simulink model "Ex4"  (R2022a)
settings: Solver=FixedStepAuto  StartTime=0.0  StopTime=5  FixedStep=0.1  RelTol=1e-3
undefined symbols (not defined in the file or in its folder): ThetaA0, XdotC0
settings Model: Creator=vfton  LastModifiedBy=vfton

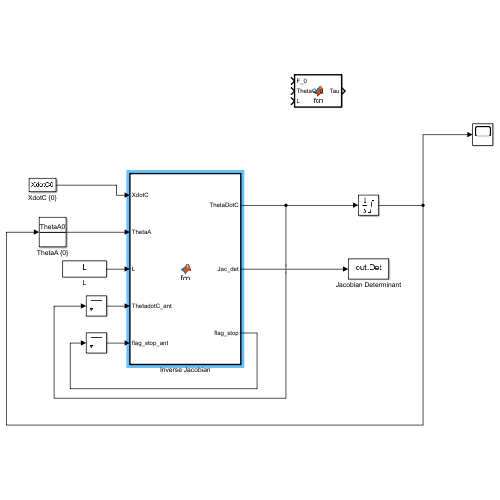
[thumbnail: Simulink's stored preview of the top-level diagram]
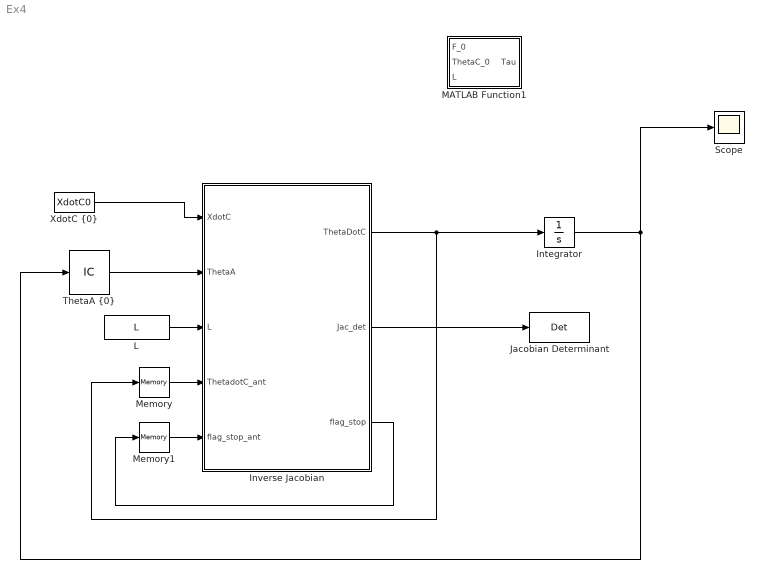
== system Ex4 ==
  Integrator : Integrator  InitialCondition=ThetaA0  LimitOutput=on  UpperSaturationLimit=[170; 170; 170]  LowerSaturationLimit=[-170;-170;-170]
  Inverse Jacobian : MATLAB Function  TreatAsAtomicUnit=on
  Jacobian Determinant : ToWorkspace  VariableName=Det  SaveFormat=Timeseries  SampleTime=-1
  L : FromWorkspace  VariableName=L
  MATLAB Function1 : MATLAB Function  TreatAsAtomicUnit=on
  Memory : Memory
  Memory1 : Memory
  Scope : Scope
  "ThetaA {0}" : InitialCondition  Value=ThetaA0
  "XdotC {0}" : Constant  Value=XdotC0
  wires:
  "XdotC {0}"/1 -> Inverse Jacobian/1(XdotC)
  L/1 -> Inverse Jacobian/3(L)
  "ThetaA {0}"/1 -> Inverse Jacobian/2(ThetaA)
  Inverse Jacobian/1(ThetaDotC) -> Memory/1, Integrator/1
  Inverse Jacobian/2(Jac_det) -> Jacobian Determinant/1
  Memory/1 -> Inverse Jacobian/4(ThetadotC_ant)
  Memory1/1 -> Inverse Jacobian/5(flag_stop_ant)
  Inverse Jacobian/3(flag_stop) -> Memory1/1
  Integrator/1 -> Scope/1, "ThetaA {0}"/1

== matlab function Ex4/MATLAB Function1 ==
  data: F_0 input; Tau output; ThetaC_0 input; L input
function Tau = fcn(F_0,ThetaC_0,L)
    Tau = 0

== matlab function Ex4/Inverse Jacobian ==
  data: ThetaDotC output; XdotC input; Jac_det output; ThetaA input; L input; ThetadotC_ant input; flag_stop_ant input; flag_stop output
function [ThetaDotC,Jac_det,flag_stop]= fcn(XdotC,ThetaA,L,ThetadotC_ant,flag_stop_ant)
    J0 = jacobian(ThetaA,L);
    J0inv = inv(J0);
    ThetaDotC = J0inv*XdotC
    Jac_det = det(J0inv);
    flag_stop = 0
